simulink model "Copy_of_diagram"  (R2025a)
settings: Solver=VariableStepAuto  StartTime=0.0  StopTime=100  RelTol=1e-3
libraries: simulink x1
settings Model: Creator=Okuyt

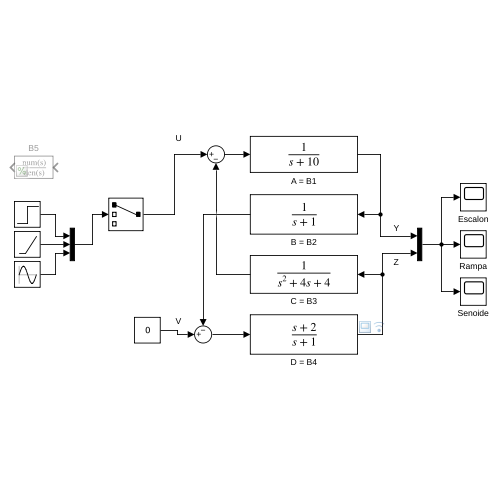
[thumbnail: Simulink's stored preview of the top-level diagram]
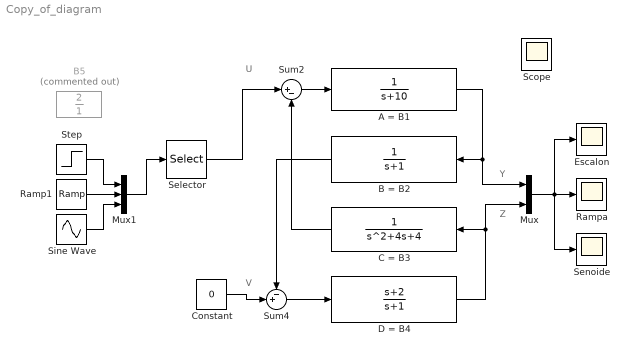
== system Copy_of_diagram ==
  note: Y
  note: Z
  note: U
  note: V
  A = B1 : TransferFcn  Denominator=[1 10]
  B = B2 : TransferFcn  Denominator=[1 1]
  B5 : TransferFcn  Commented=on  Numerator=[2]  Denominator=[1]
  C = B3 : TransferFcn  Denominator=[1 4 4]
  Constant : Constant  Value=0
  D = B4 : TransferFcn  Numerator=[1 2]  Denominator=[1 1]
  Escalon : Scope
      settings: TimeSpan=100  ActiveDisplayYMinimum=-0.2  ActiveDisplayYMaximum=2.2  DataLoggingVariableName=ScopeData3
  Mux : Mux  Inputs=2
  Mux1 : Mux  Inputs=3
  Ramp1 : simulink/Sources/Ramp  slope=1  start=0  InitialOutput=0
  Rampa : Scope
      settings: TimeSpan=100  ActiveDisplayYMinimum=-0.29997  ActiveDisplayYMaximum=0.2
  Selector : Selector  InputPortWidth=3  IndexOptions=Index vector (dialog)  Indices=1  OutputSizes=1
  Senoide : Scope
      settings: TimeSpan=100  ActiveDisplayYMinimum=-1.5  ActiveDisplayYMaximum=1.5  DataLoggingVariableName=ScopeData2
  Sine Wave : Sin  SampleTime=0
  Step : Step  SampleTime=0
  Sum2 : Sum  Inputs=|+-
  Sum4 : Sum  Inputs=-+|
  Scope : Scope
      settings: ActiveDisplayYMinimum=-7.96675  ActiveDisplayYMaximum=13.90038
  wires:
  Mux/1 -> Escalon/1, Rampa/1, Senoide/1
  Mux1/1 -> Selector/1
  Step/1 -> Mux1/1
  Ramp1/1 -> Mux1/2
  Sine Wave/1 -> Mux1/3
  Sum2/1 -> A = B1/1
  B = B2/1 -> Sum4/1
  C = B3/1 -> Sum2/2
  A = B1/1 -> B = B2/1, Mux/1
  D = B4/1 -> C = B3/1, Mux/2
  Sum4/1 -> D = B4/1
  Constant/1 -> Sum4/2
  Selector/1 -> Sum2/1
